simulink model "ttc_ut"  (Simulink 8.1)
settings: Solver=FixedStepDiscrete  StartTime=0.0  StopTime=10.0  FixedStep=0.005  RelTol=1e-3
libraries: siltestlib x20, ttc x1
settings Model: Creator=xsellart  LastModifiedBy=AT015555
settings DataIOCC: SignalLoggingSaveFormat=Dataset
settings OptimizationCC: ExpressionDepthLimit=128
settings DebuggingCC: FcnCallInpInsideContextMsg=EnableAllAsError
settings GRTTargetCC: CombineOutputUpdateFcns=on  GRTInterface=off

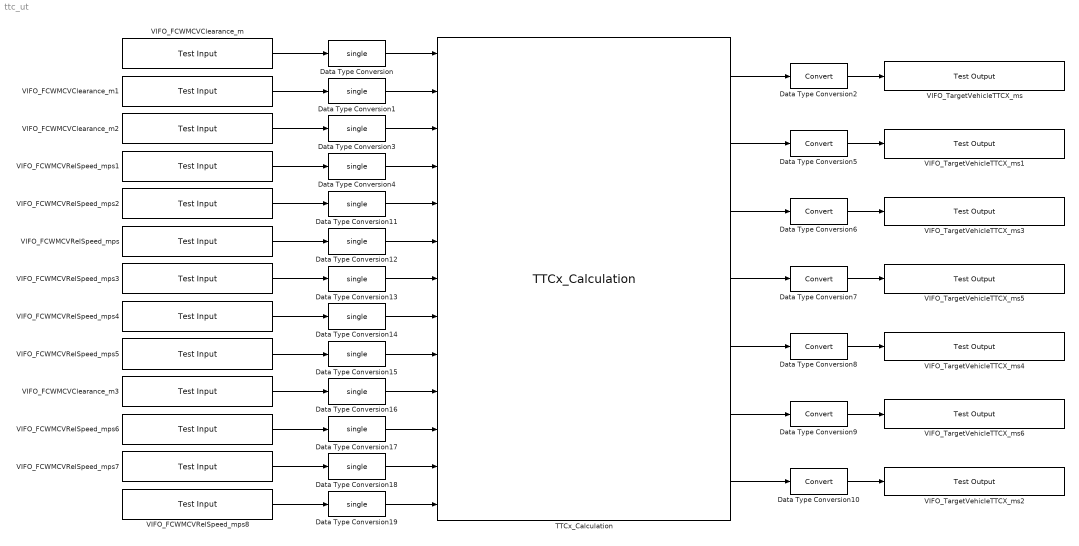
== system ttc_ut ==
  Data Type Conversion{,1,3..4,11..19} (13 alike) : DataTypeConversion  OutDataTypeStr=single
  Data Type Conversion{2,5..10} (7 alike) : DataTypeConversion
  TTCx_Calculation : ttc/TTCx_Calculation
  VIFO_FCWMCVClearance_m : siltestlib/Test Input  varname=VIFO_FCWMCVehXPosition_m  sampletime=0.005
  VIFO_FCWMCVClearance_m1 : siltestlib/Test Input  varname=VIFO_AEBMCVehXPosition_m  sampletime=0.005
  VIFO_FCWMCVClearance_m2 : siltestlib/Test Input  varname=VIFO_ACCMCVehXPosition_m  sampletime=0.005
  VIFO_FCWMCVClearance_m3 : siltestlib/Test Input  varname=VIFO_VRUMCPedXPosition_m  sampletime=0.005
  VIFO_FCWMCVRelSpeed_mps : siltestlib/Test Input  varname=VIFO_ACCTargetVehRelSpeedX_mps  sampletime=0.005
  VIFO_FCWMCVRelSpeed_mps1 : siltestlib/Test Input  varname=VIFO_FCWTargetVehRelSpeedX_mps  sampletime=0.005
  VIFO_FCWMCVRelSpeed_mps2 : siltestlib/Test Input  varname=VIFO_AEBTargetVehRelSpeedX_mps  sampletime=0.005
  VIFO_FCWMCVRelSpeed_mps3 : siltestlib/Test Input  varname=VIFO_FCWMCLongAcc_mps2  sampletime=0.005
  VIFO_FCWMCVRelSpeed_mps4 : siltestlib/Test Input  varname=VIFO_AEBMCLongAcc_mps2  sampletime=0.005
  VIFO_FCWMCVRelSpeed_mps5 : siltestlib/Test Input  varname=VIFO_ACCMCLongAcc_mps2  sampletime=0.005
  VIFO_FCWMCVRelSpeed_mps6 : siltestlib/Test Input  varname=VIFO_VRUMCLongAcc_mps2  sampletime=0.005
  VIFO_FCWMCVRelSpeed_mps7 : siltestlib/Test Input  varname=VIFO_VRUTargetPedRelSpeedX_mps  sampletime=0.005
  VIFO_FCWMCVRelSpeed_mps8 : siltestlib/Test Input  varname=VDINR_LongAcc_G  sampletime=0.005
  VIFO_TargetVehicleTTCX_ms : siltestlib/Test Output  varname=VIFO_FCWVehClearance_m  sampletime=-1
  VIFO_TargetVehicleTTCX_ms1 : siltestlib/Test Output  varname=VIFO_FCWTargetVehicleTtcX_ms  sampletime=-1
  VIFO_TargetVehicleTTCX_ms2 : siltestlib/Test Output  varname=VIFO_AEBVehClearance_m  sampletime=-1
  VIFO_TargetVehicleTTCX_ms3 : siltestlib/Test Output  varname=VIFO_AEBTargetVehicleTtcX_ms  sampletime=-1
  VIFO_TargetVehicleTTCX_ms4 : siltestlib/Test Output  varname=VIFO_VRUPedClearance_m  sampletime=-1
  VIFO_TargetVehicleTTCX_ms5 : siltestlib/Test Output  varname=VIFO_ACCTargetVehicleTtcX_ms  sampletime=-1
  VIFO_TargetVehicleTTCX_ms6 : siltestlib/Test Output  varname=VIFO_VRUTargetPedTtcX_ms  sampletime=-1
  wires:
  VIFO_FCWMCVClearance_m/1 -> Data Type Conversion/1
  VIFO_FCWMCVClearance_m1/1 -> Data Type Conversion1/1
  Data Type Conversion1/1 -> TTCx_Calculation/2
  TTCx_Calculation/1 -> Data Type Conversion2/1
  Data Type Conversion2/1 -> VIFO_TargetVehicleTTCX_ms/1
  Data Type Conversion/1 -> TTCx_Calculation/1
  VIFO_FCWMCVClearance_m2/1 -> Data Type Conversion3/1
  VIFO_FCWMCVRelSpeed_mps1/1 -> Data Type Conversion4/1
  Data Type Conversion4/1 -> TTCx_Calculation/4
  Data Type Conversion3/1 -> TTCx_Calculation/3
  TTCx_Calculation/2 -> Data Type Conversion5/1
  Data Type Conversion5/1 -> VIFO_TargetVehicleTTCX_ms1/1
  TTCx_Calculation/3 -> Data Type Conversion6/1
  Data Type Conversion6/1 -> VIFO_TargetVehicleTTCX_ms3/1
  TTCx_Calculation/4 -> Data Type Conversion7/1
  Data Type Conversion7/1 -> VIFO_TargetVehicleTTCX_ms5/1
  Data Type Conversion8/1 -> VIFO_TargetVehicleTTCX_ms4/1
  TTCx_Calculation/5 -> Data Type Conversion8/1
  TTCx_Calculation/6 -> Data Type Conversion9/1
  Data Type Conversion9/1 -> VIFO_TargetVehicleTTCX_ms6/1
  TTCx_Calculation/7 -> Data Type Conversion10/1
  Data Type Conversion10/1 -> VIFO_TargetVehicleTTCX_ms2/1
  VIFO_FCWMCVRelSpeed_mps2/1 -> Data Type Conversion11/1
  Data Type Conversion11/1 -> TTCx_Calculation/5
  VIFO_FCWMCVRelSpeed_mps/1 -> Data Type Conversion12/1
  Data Type Conversion12/1 -> TTCx_Calculation/6
  VIFO_FCWMCVRelSpeed_mps3/1 -> Data Type Conversion13/1
  VIFO_FCWMCVRelSpeed_mps4/1 -> Data Type Conversion14/1
  VIFO_FCWMCVRelSpeed_mps5/1 -> Data Type Conversion15/1
  VIFO_FCWMCVClearance_m3/1 -> Data Type Conversion16/1
  VIFO_FCWMCVRelSpeed_mps6/1 -> Data Type Conversion17/1
  VIFO_FCWMCVRelSpeed_mps7/1 -> Data Type Conversion18/1
  VIFO_FCWMCVRelSpeed_mps8/1 -> Data Type Conversion19/1
  Data Type Conversion13/1 -> TTCx_Calculation/7
  Data Type Conversion14/1 -> TTCx_Calculation/8
  Data Type Conversion18/1 -> TTCx_Calculation/12
  Data Type Conversion19/1 -> TTCx_Calculation/13
  Data Type Conversion15/1 -> TTCx_Calculation/9
  Data Type Conversion17/1 -> TTCx_Calculation/11
  Data Type Conversion16/1 -> TTCx_Calculation/10
